simulink model "Figure_2_1_TP_Telecom_modulationask2"  (R2020a)
settings: Solver=VariableStepAuto  StartTime=0.0  StopTime=10  RelTol=1e-3
libraries: commrandsrc3 x1, dspsigops x1, commutil2 x1, dspsrcs4 x1
Description:
  | C'est un TP Télécom à faire.
settings Model: Creator=Mr Ibrahima BA  LastModifiedBy=iba

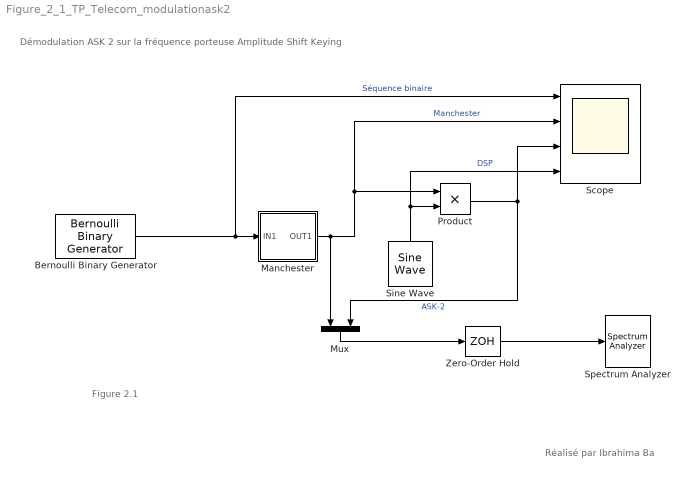
== system Figure_2_1_TP_Telecom_modulationask2 ==
  note: Réalisé par Ibrahima Ba
  note: Démodulation ASK 2 sur la fréquence porteuse
      | Amplitude Shift Keying
  note: Figure 2.1
  "Bernoulli Binary Generator " : commrandsrc3/Bernoulli Binary Generator  ProbabilityOfZero=0.5  SeedSource=Parameter  Seed=25.  SampleTime=1  SamplesPerFrame=1  OutputDataType=double  SimulateUsing=Interpreted execution
  Manchester : Subsystem
  Mux : Mux  Inputs=2
  "Product " : Product  OutDataTypeStr=double  LockScale=on
  "Scope " : Scope  NumInputPorts=4
  Sine Wave : dspsrcs4/Sine Wave  Amplitude=1  Frequency=5  Phase=0  SampleMode=Discrete  OutComplex=Real  CompMethod=Trigonometric fcn  TableSize=Speed  SampleTime=1/1000  SamplesPerFrame=1  ResetState=Restart at time zero  OutputFrames=off  dataType=Inherit via back propagation  wordLen=16  udDataType=sfix(16)  fracBitsMode=Best precision  numFracBits=15  OutDataTypeStr=Inherit: Inherit via back propagation  LastOutDataTypeStr=Inherit: Inherit via back propagation
  "Spectrum Analyzer " : SpectrumAnalyzer
  "Zero-Order Hold " : ZeroOrderHold  SampleTime=0.05
  wires:
  "Bernoulli Binary Generator "/1 -> "Scope "/1, Manchester/1(IN1)  "Séquence binaire"
  Manchester/1(OUT1) -> "Scope "/2, "Product "/1, Mux/1  "Manchester"
  "Zero-Order Hold "/1 -> "Spectrum Analyzer "/1
  "Product "/1 -> Mux/2, "Scope "/3  "ASK-2"
  Mux/1 -> "Zero-Order Hold "/1
  Sine Wave/1 -> "Scope "/4, "Product "/2  "DSP"

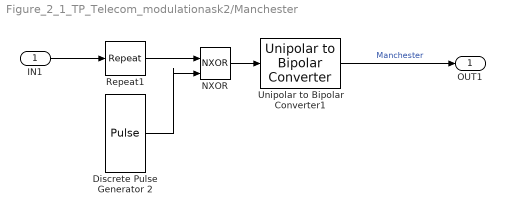
== system Figure_2_1_TP_Telecom_modulationask2/Manchester ==
  IN1 : Inport
  "Discrete Pulse Generator 2  " : DiscretePulseGenerator  SampleTime=0.5
  "NXOR " : Logic  Operator=NXOR  IconShape=distinctive  AllPortsSameDT=off  OutDataTypeStr=boolean
  Repeat1 : dspsigops/Repeat  N=2  InputProcessing=Columns as channels (frame based)  RateOptions=Enforce single-rate processing  ic=0  mode=Unused parameter value
  Unipolar to Bipolar Converter1 : commutil2/Unipolar to Bipolar Converter  M=2  polarity=Positive  dataType=double
  OUT1 : Outport
  wires:
  IN1/1 -> Repeat1/1
  "NXOR "/1 -> Unipolar to Bipolar Converter1/1
  "Discrete Pulse Generator 2  "/1 -> "NXOR "/2
  Unipolar to Bipolar Converter1/1 -> OUT1/1  "Manchester"
  Repeat1/1 -> "NXOR "/1
